simulink model "anfis_test"  (R2017b)
settings: Solver=VariableStepAuto  StartTime=0.0  StopTime=10.0  RelTol=1e-3
values from neighbouring files (symbols this model uses):
  coeff_sim = [0.05 306.39 0.001]    [ANFIS.mat]    (also in road_anfis.m = road_coeff(i+1,:))
libraries: fuzblock x1, simulink x1
settings Model: Creator=hadlaczkyb  LastModifiedBy=hadlaczkyb
settings DataIOCC: SaveFormat=Array

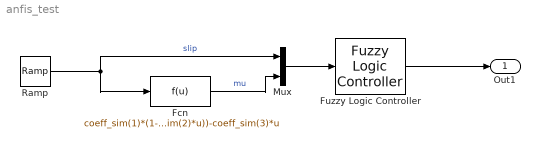
== system anfis_test ==
  Fcn : Fcn  Expr=coeff_sim(1)*(1-exp(-coeff_sim(2)*u))-coeff_sim(3)*u
  Fuzzy Logic Controller : fuzblock/Fuzzy Logic  Controller  FIS=train_fis  OutputSampleNumber=101  DataType=double  FuzzifiedInputs=off  RuleFiringStrengths=off  RuleOutputs=off  AggregatedOutputs=off  SimulateUsing=Interpreted execution
  Mux : Mux  Inputs=2
  Ramp : simulink/Sources/Ramp  slope=0.1  start=0  X0=0.1
  Out1 : Outport
  wires:
  Ramp/1 -> Mux/1, Fcn/1  "slip"
  Mux/1 -> Fuzzy Logic Controller/1
  Fuzzy Logic Controller/1 -> Out1/1
  Fcn/1 -> Mux/2  "mu"
